simulink model "rigid_body_fdyn_rotmat_test_eulangrpy"  (Simulink 8.5)
settings: Solver=ode4  StartTime=0.0  StopTime=10.0  FixedStep=1.000000e-04  RelTol=1e-3
undefined symbols (not defined in the file or in its folder): m
libraries: rigid_body_kinematics x3, rigid_body_dynamics x2, lib_rigidbody_dynamics_mapletb_mod x2
settings Model: Creator=schappler  LastModifiedBy=schappler
settings DataIOCC: LimitDataPoints=off  SaveFormat=StructureWithTime  SignalLoggingSaveFormat=Dataset
settings OptimizationCC: ExpressionDepthLimit=128
settings DebuggingCC: UnderspecifiedInitializationDetection=Simplified  MergeDetectMultiDrivingBlocksExec=error  FcnCallInpInsideContextMsg=EnableAllAsError  StateNameClashWarn=none
settings GRTTargetCC: CombineOutputUpdateFcns=on  GRTInterface=off

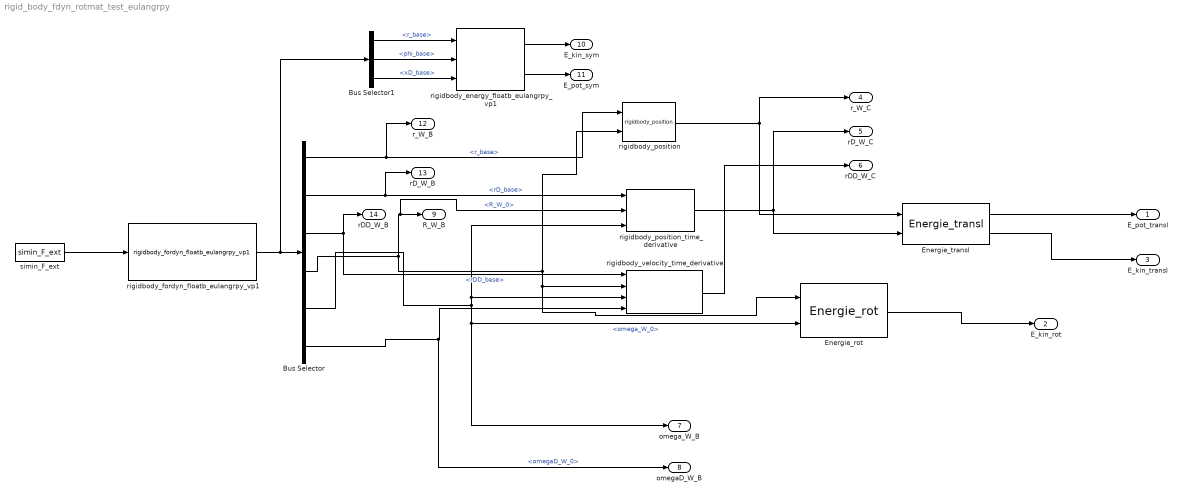
== system rigid_body_fdyn_rotmat_test_eulangrpy ==
  Bus Selector : BusSelector  OutputSignals=r_base,rD_base,rDD_base,R_W_0,omega_W_0,omegaD_W_0
  Bus Selector1 : BusSelector  OutputSignals=r_base,phi_base,xD_base
  Energie_rot : rigid_body_dynamics/Energie_rot  I_B_C=I_B_C
  Energie_transl : rigid_body_dynamics/Energie_transl  m=m  g_W=g_W
  rigidbody_energy_floatb_eulangrpy_vp1 : lib_rigidbody_dynamics_mapletb_mod/rigidbody_energy_floatb_eulangrpy_vp1  KinPar_mdh=KinPar_mdh  DynPar1=DynPar1  g_world=g_W
  rigidbody_fordyn_floatb_eulangrpy_vp1 : lib_rigidbody_dynamics_mapletb_mod/rigidbody_fordyn_floatb_eulangrpy_vp1  r_base_t0=r0  rD_base_t0=rD0  phi_base_t0=phi_base_t0  phiD_base_t0=phiD_base_t0  g_world=g_W  KinPar_mdh=KinPar_mdh  DynPar1=DynPar1
  rigidbody_position : rigid_body_kinematics/rigidbody_position  r_B_B_C=r_B_B_C  PktName_B='B'  PktName_C='C'
  rigidbody_position_time_derivative : rigid_body_kinematics/rigidbody_position_time_derivative  r_B_B_C=r_B_B_C  PktName_B='B'  PktName_C='C'
  rigidbody_velocity_time_derivative : rigid_body_kinematics/rigidbody_velocity_time_derivative  r_B_B_C=r_B_B_C  PktName_B='B'  PktName_C='C'
  simin_F_ext : FromWorkspace  VariableName=simin_F_ext  SampleTime=0  Interpolate=off  OutputAfterFinalValue=Holding final value
  E_pot_transl : Outport
  E_kin_rot : Outport  Port=2
  E_kin_transl : Outport  Port=3
  r_W_C : Outport  Port=4
  rD_W_C : Outport  Port=5
  rDD_W_C : Outport  Port=6
  omega_W_B : Outport  Port=7
  omegaD_W_B : Outport  Port=8
  R_W_B : Outport  Port=9
  E_kin_sym : Outport  Port=10
  E_pot_sym : Outport  Port=11
  r_W_B : Outport  Port=12
  rD_W_B : Outport  Port=13
  rDD_W_B : Outport  Port=14
  wires:
  rigidbody_position/1 -> Energie_transl/1, r_W_C/1
  rigidbody_position_time_derivative/1 -> rD_W_C/1, Energie_transl/2
  rigidbody_velocity_time_derivative/1 -> rDD_W_C/1
  Energie_transl/1 -> E_pot_transl/1
  Energie_transl/2 -> E_kin_transl/1
  Energie_rot/1 -> E_kin_rot/1
  rigidbody_fordyn_floatb_eulangrpy_vp1/1 -> Bus Selector1/1, Bus Selector/1
  Bus Selector/1 -> rigidbody_position/1, r_W_B/1  "<r_base>"
  Bus Selector/3 -> rDD_W_B/1, rigidbody_velocity_time_derivative/1  "<rDD_base>"
  Bus Selector/5 -> omega_W_B/1, Energie_rot/2, rigidbody_position_time_derivative/3, rigidbody_velocity_time_derivative/3  "<omega_W_0>"
  Bus Selector/6 -> rigidbody_velocity_time_derivative/4, omegaD_W_B/1  "<omegaD_W_0>"
  Bus Selector/2 -> rigidbody_position_time_derivative/1, rD_W_B/1  "<rD_base>"
  Bus Selector/4 -> rigidbody_position/2, rigidbody_velocity_time_derivative/2, Energie_rot/1, rigidbody_position_time_derivative/2, R_W_B/1  "<R_W_0>"
  rigidbody_energy_floatb_eulangrpy_vp1/1 -> E_kin_sym/1
  rigidbody_energy_floatb_eulangrpy_vp1/2 -> E_pot_sym/1
  Bus Selector1/3 -> rigidbody_energy_floatb_eulangrpy_vp1/3  "<xD_base>"
  Bus Selector1/1 -> rigidbody_energy_floatb_eulangrpy_vp1/1  "<r_base>"
  Bus Selector1/2 -> rigidbody_energy_floatb_eulangrpy_vp1/2  "<phi_base>"
  simin_F_ext/1 -> rigidbody_fordyn_floatb_eulangrpy_vp1/1
